simulink model "untitled"  (R2020b)
settings: Solver=VariableStepAuto  StartTime=0.0  StopTime=10.0  RelTol=1e-3
settings Model: Creator=phar0732  LastModifiedBy=phar0732
settings DataIOCC: LimitDataPoints=on  SaveOutput=off  SaveTime=off
settings OptimizationCC: BlockReduction=off  BooleanDataType=off  LifeSpan=inf
settings DebuggingCC: SaveWithParameterizedLinksMsg=none  UnderspecifiedInitializationDetection=Classic  MergeDetectMultiDrivingBlocksExec=none  SignalResolutionControl=TryResolveAllWithWarning  AllowSymbolicDim=off  SFUnexpectedBacktrackingDiag=warning  SFNoUnconditionalDefaultTransitionDiag=warning  SFExecutionAtInitializationDiag=none  ArithmeticOperatorsInVariantConditions=warning
settings HardwareCC: TargetUnknown=on
settings SFSimCC: SimUseLocalCustomCode=off  CustomCodeUndefinedFunction=UseInterfaceOnly
settings RTWCC: RTWUseLocalCustomCode=off
settings CodeAppCC: StateflowObjectComments=on
settings GRTTargetCC: TargetLangStandard=C89/C90 (ANSI)

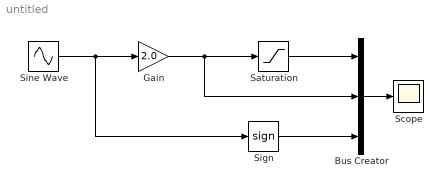
== system untitled ==
  Bus Creator : BusCreator  Inputs=3
  Gain : Gain  Gain=2.0
  Saturation : Saturate
  Scope : Scope
  Sign : Signum
  Sine Wave : Sin  SampleTime=0
  wires:
  Gain/1 -> Bus Creator/2, Saturation/1
  Sine Wave/1 -> Sign/1, Gain/1
  Bus Creator/1 -> Scope/1
  Saturation/1 -> Bus Creator/1
  Sign/1 -> Bus Creator/3
